simulink model "testmodell"  (R2016b)
settings: Solver=VariableStepAuto  StartTime=0.0  StopTime=10.0  RelTol=1e-3
libraries: simulink x1
settings Model: Creator=ga35gug  LastModifiedBy=ga35gug

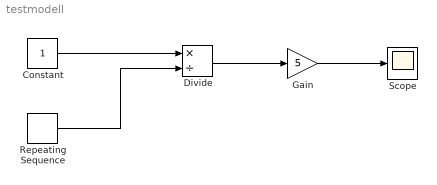
== system testmodell ==
  Constant : Constant
  Divide : Product  Inputs=*/
  Gain : Gain  Gain=5
  Repeating Sequence : simulink/Sources/Repeating Sequence  rep_seq_t=[0 2]  rep_seq_y=[0 2]
  Scope : Scope
  wires:
  Constant/1 -> Divide/1
  Repeating Sequence/1 -> Divide/2
  Divide/1 -> Gain/1
  Gain/1 -> Scope/1
